simulink model "HVDC_MMC1_EMT"  (R2023b)
settings: Solver=ode23tb  StartTime=0.0  StopTime=10  MaxStep=Ts  RelTol=1e-3  EnableMultiTasking=on
PreLoadFcn:
  | HVDC_MMC_param
StartFcn:
  | tic
StopFcn:
  | toc
values from neighbouring files (symbols this model uses):
  acdcV = 1/(Vnom_dc/2*sqrt(3)/sqrt(2)/Vnom_sec)    [HVDC_MMC_param.m]
  C_PM = 1.758e-3    (= 0.001758)    [HVDC_MMC_param.m]
  Carm = 1.0*C_pm/n    (= 0.0002096)    [B2B_HVDC_MMC_Calc.m]    (also in HVDC_MMC_param.m = 4.88333333333e-05)
  DC_cable_C_shunt = 0.1e-6    (= 1e-07)    [HVDC_MMC_param.m]
  DC_cable_R_shunt = 1000    [HVDC_MMC_param.m]
  DCM = 1    [HVDC_MMC_param.m]
  Fn_filter = 1000    [B2B_HVDC_MMC_Calc.m]    (also in HVDC_MMC_param.m)
  Fnom = 50    [HVDC_MMC_param.m]
  HRM = 2    [HVDC_MMC_param.m]
  HrmOrd = N    (= 2)    [B2B_HVDC_MMC_Calc.m]    (also in HVDC_MMC_param.m)
  Ib_ac = (2/3)*Pnom/Vb_ac    [HVDC_MMC_param.m]
  Ib_dc = Pnom/Vb_dc    (= 1501.5015015)    [HVDC_MMC_param.m]
  Ki_CCSC = 50    [HVDC_MMC_param.m]
  Ki_Ireg = 6    [HVDC_MMC_param.m]
  Ki_Preg = 1.0    (= 1)    [HVDC_MMC_param.m]
  Ki_Qreg = 1.0    (= 1)    [HVDC_MMC_param.m]
  Ki_VDCreg = 100    [HVDC_MMC_param.m]
  Kp_CCSC = 0.8    [HVDC_MMC_param.m]
  Kp_Ireg = 0.6    [HVDC_MMC_param.m]
  Kp_Preg = 0.5/3    (= 0.166666666667)    [HVDC_MMC_param.m]
  Kp_Qreg = 0.5/3    (= 0.166666666667)    [HVDC_MMC_param.m]
  Kp_VDCreg = 4    [HVDC_MMC_param.m]
  L_cable = 15e-3    (= 0.015)    [HVDC_MMC_param.m]
  Larm = Larm_pu*(Zb_ac/w)    [HVDC_MMC_param.m]
  Lff = Larm_pu/2+Lxfo    (= 0.195)    [HVDC_MMC_param.m]
  Limits_Ireg = [ 2.0  -2.0]    [HVDC_MMC_param.m]
  Limits_Preg = [ 1.2, 0.8 ]    [HVDC_MMC_param.m]
  Limits_Qreg = [ 0.25, -0.25 ]    [HVDC_MMC_param.m]
  Limits_VDCreg = [ 2.0  -2.0]    [HVDC_MMC_param.m]
  Lxfo = 0.12    [HVDC_MMC_param.m]
  Pac = 0.9    [HVDC_MMC_param.m]
  Pnom = 1000e6    (= 1000000000)    [HVDC_MMC_param.m]
  Qac = 0.2    [HVDC_MMC_param.m]
  QCM = 0    [HVDC_MMC_param.m]
  R_cable = 0.5    [HVDC_MMC_param.m]
  Rarm = Rarm_pu*Zb_ac    [HVDC_MMC_param.m]
  Rff = Rarm_pu/2+Rxfo    (= 0.00375)    [HVDC_MMC_param.m]
  Rxfo = 0.003    [HVDC_MMC_param.m]
  Slope_Pref = 0.5    [HVDC_MMC_param.m]
  Slope_Qref = 0.5    [HVDC_MMC_param.m]
  Slope_Vdc_ref = Vnom_dc/5    (= 133200)    [HVDC_MMC_param.m]
  Tbrk1_On = 0.1    [HVDC_MMC_param.m]
  Tbrk2_On = 1.0    (= 1)    [HVDC_MMC_param.m]
  Tdeblock = 1.5    [HVDC_MMC_param.m]
  Tfault = 9999    [HVDC_MMC_param.m]
  Ton_Converter2 = 3    [HVDC_MMC_param.m]
  Ton_PQreg = 2    [HVDC_MMC_param.m]
  Ton_VDCreg = 1.5    [HVDC_MMC_param.m]
  Ts = Ts_Power    (= 5e-05)    [B2B_HVDC_MMC_Calc.m]    (also in HVDC_MMC_param.m)
  Ts_Control = Ts_Power    (= 5e-05)    [B2B_HVDC_MMC_Calc.m]    (also in HVDC_MMC_param.m)
  Ts_DQN = MultTs*Ts_Power    (= 5e-05)    [B2B_HVDC_MMC_Calc.m]    (also in HVDC_MMC_param.m)
  Ts_EMT = Ts    (= 5e-05)    [HVDC_MMC_param.m]
  Ts_Power = 1*50e-6    (= 5e-05)    [B2B_HVDC_MMC_Calc.m]    (also in HVDC_MMC_param.m)
  Vb_ac = sqrt(2/3)*Vnom_sec    [HVDC_MMC_param.m]
  Vb_dc = Vnom_dc    (= 666000)    [HVDC_MMC_param.m]
  Vc0_PM = 0    [HVDC_MMC_param.m]
  Vnom_dc = 2*Vnom_sec    (= 666000)    [HVDC_MMC_param.m]
  Vnom_prim = 333e3    (= 333000)    [HVDC_MMC_param.m]
  Vnom_sec = 333e3    (= 333000)    [HVDC_MMC_param.m]
  w = 2*pi*f    (= 314.159265359)    [B2B_HVDC_MMC_Calc.m]    (also in HVDC_MMC_param.m)
  Ws = 2*pi*Fnom    (= 314.159265359)    [HVDC_MMC_param.m]
  Zb_ac = Vb_ac/Ib_ac    [HVDC_MMC_param.m]
  Zeta_filter = 1    [B2B_HVDC_MMC_Calc.m]    (also in HVDC_MMC_param.m)
undefined symbols (not defined in the file or in its folder): DCss, DiscIntNeverNeededParam, gcbh, MT, sps_rtmsupport
libraries: DQN_Lib x37, simulink x35, spsCurrentMeasurementLib x24, powerlib_extras x21, slpidlib x14, spsSecondOrderFilterLib x14, spsVoltageMeasurementLib x10, spsSeriesRLCBranchLib x10, spsControlledVoltageSourceLib x9, spsHalfBridgeMMCmodel x7, spsGroundLib x4, spsParallelRLCBranchLib x4
(part 3 of 9)

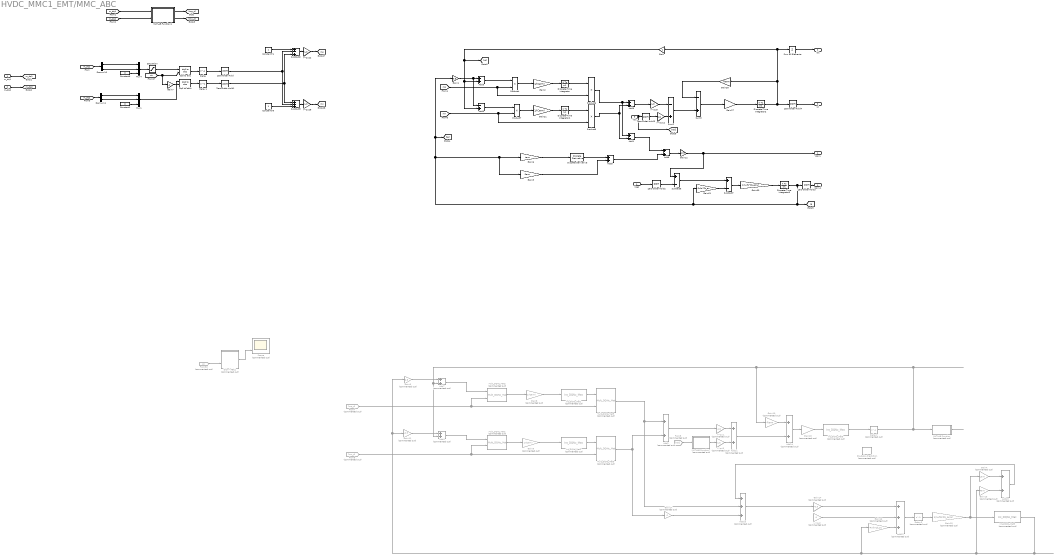
== system HVDC_MMC1_EMT/MMC_ABC ==
  m_dq1 : Inport
  m_dq2 : Inport  Port=2
  Vdc : Inport  Port=3
  Vsec : Inport  Port=4
  Add1 : Sum  Inputs=+-
  Add10 : Sum  Commented=on  Inputs=+++
  Add{2,4,7,11,13..14} (6 alike) : Sum  Commented=on
  Add12 : Sum  Commented=on  Inputs=+++
  Add{3,5,8..9} (4 alike) : Sum
  Add6 : Sum  Inputs=-+
  Constant1 : Constant  Value=0
  Constant6 : Constant  Value=0
  Constant74 : Constant
  Constant75 : Constant
  DQn->ABC1 : MATLAB Function  Commented=on  TreatAsAtomicUnit=on  SystemSampleTime=Ts  mask{N=HrmOrd}
      mask prompts: N "Harmonic order:"
  Delay : Delay  DelayLength=1
  Delay1 : Delay  DelayLength=1
  Delay2 : Delay  Commented=on  DelayLength=1  SampleTime=Ts
  Delay3 : Delay  Commented=on  DelayLength=1  SampleTime=Ts
  Demux10 : Demux  Outputs=2
  Demux11 : Demux  Outputs=2
  Discrete Derivative : simulink/Discrete/Discrete Derivative  gainval=1.0  ICPrevScaledInput=0.0  OutMin=[]  OutMax=[]  OutDataType=fixdt(1, 16)  OutScaling=2^-10  DoSatur=off
  Discrete-Time Integrator{,1..3} (4 alike) : DiscreteIntegrator  SampleTime=Ts_EMT  ICPrevOutput=DiscIntNeverNeededParam  ICPrevScaledInput=DiscIntNeverNeededParam
  From30 : From  Commented=on  GotoTag=wt  TagVisibility=global
  From5 : From  Commented=on  GotoTag=Vdc
  From7 : From  Commented=on  GotoTag=mp_c
  From8 : From  Commented=on  GotoTag=mn_c
  Gain : Gain
  Gain1 : Gain  Gain=0.5
  Gain10 : Gain  Commented=on  Gain=-Rarm
  Gain11 : Gain  Commented=on  Gain=-0.5
  Gain12 : Gain  Gain=-0.5
  Gain13 : Gain  Commented=on  Gain=Rarm
  Gain14 : Gain  Commented=on  Gain=-0.5
  Gain15 : Gain  Commented=on  Gain=1/(Lxfo*Zb_ac/w)
  Gain16 : Gain  Commented=on  Gain=-Rxfo*Zb_ac
  Gain17 : Gain  Commented=on  Gain=-1
  Gain18 : Gain  Commented=on  Gain=1/(Larm)
  Gain2 : Gain  Gain=1/(Carm)
  Gain21 : Gain  Gain=1/(Carm)
  Gain27 : Gain  Gain=1/(Larm)
  Gain28 : Gain  Gain=Rarm
  Gain3 : Gain  Gain=Rarm
  Gain4 : Gain  Commented=on  Gain=Larm
  Gain5 : Gain  Commented=on  Gain=0.5
  Gain6 : Gain  Gain=Larm
  Gain60 : Gain  Gain=1/(Lxfo*Zb_ac/w)
  Gain61 : Gain  Gain=Rxfo*Zb_ac
  Gain7 : Gain  Gain=-2
  Gain8 : Gain  Commented=on  Gain=1/(Carm)
  Gain9 : Gain  Commented=on  Gain=1/(Carm)
  I->pu1 : Gain  Commented=on  Gain=-1/2  SaturateOnIntegerOverflow=on  OutDataTypeStr=Inherit: Same as input  ParamDataTypeStr=Inherit: Same as input
  I->pu{5,12,22,28} (4 alike) : Gain  Gain=1/2  SaturateOnIntegerOverflow=on  OutDataTypeStr=Inherit: Same as input  ParamDataTypeStr=Inherit: Same as input
  I->pu2 : Gain  Commented=on  Gain=-1  SaturateOnIntegerOverflow=on  OutDataTypeStr=Inherit: Same as input  ParamDataTypeStr=Inherit: Same as input
  I->pu3 : Gain  Commented=on  Gain=1/2  SaturateOnIntegerOverflow=on  OutDataTypeStr=Inherit: Same as input  ParamDataTypeStr=Inherit: Same as input
  Int_DQNc_Mat{1..3,5} (4 alike) : DQN_Lib/Int_DQNc_Mat  Commented=on  N=HrmOrd  dt=Ts  w=Ws  InitInt=0*[0.8; 0.6; -0.33]  swFeed=off  R=1  iL=1
  MATLAB Function : MATLAB Function  Commented=on  TreatAsAtomicUnit=on
  MATLAB Function1 : MATLAB Function  TreatAsAtomicUnit=on  mask{N=HrmOrd}
      mask prompts: N "Harmonic order:"
  MATLAB Function2 : MATLAB Function  Commented=on  TreatAsAtomicUnit=on  mask{N=HrmOrd}
      mask prompts: N "Harmonic order:"
  Mult_DQNc_Mat{1..3,5} (4 alike) : DQN_Lib/Mult_DQNc_Mat  Commented=on  N=HrmOrd  HrmDbl=off
  Mux1 : Mux  Inputs=3
  Mux4 : Mux  Inputs=3
  Product{4,6..8} (4 alike) : Product
  SS_DelayPrediction : DQN_Lib/SS_DelayPrediction  Commented=on  N=HrmOrd  Ts=Ts  x0=zeros(3,1)
  Saturation : Saturate  UpperLimit=Limits_Ireg(1)  LowerLimit=Limits_Ireg(2)
  Scope : Scope  Commented=on  NumInputPorts=2
  Subtract2 : Sum  Inputs=+-+
  Subtract5 : Sum  Inputs=+++
  Subtract6 : Sum  Inputs=+-
  Subtract7 : Sum  Inputs=+-
  Sum of Elements : Sum  Inputs=+
  Sum2 : Sum  Inputs=-+  InputSameDT=on  SaturateOnIntegerOverflow=on  OutDataTypeStr=Inherit: Same as first input
  Sum3 : Sum  Inputs=-+  InputSameDT=on  SaturateOnIntegerOverflow=on  OutDataTypeStr=Inherit: Same as first input
  Zero-Order Hold{,1..3} (4 alike) : ZeroOrderHold  SampleTime=Ts_EMT
  Zero-Order Hold4 : ZeroOrderHold  SampleTime=Ts
  Zero-Order Hold5 : ZeroOrderHold  SampleTime=Ts
  dq0 to abc : spsdq0toabcLib/dq0 to abc  Alignment=90 degrees behind phase A axis
  dq0 to abc1 : spsdq0toabcLib/dq0 to abc  Alignment=90 degrees behind phase A axis
  Vconv : Outport
  Idc : Outport  Port=2
  Id : Outport  Port=3
  Iconv1 : Outport  Port=4  VectorParamsAs1DForOutWhenUnconnected=off
  tag scope: Ig=global, m_dq1=global, m_dq2=global, mn=global, mp=global
  wires:
  Gain21/1 -> Discrete-Time Integrator1/1  "dVn_M"
  Add6/1 -> Product7/1
  Discrete-Time Integrator2/1 -> Zero-Order Hold4/1, Gain/1, Sum of Elements/1, Gain28/1  "dVp_M"
  Gain1/1 -> Add6/1, Add3/1
  Sum2/1 -> Sum3/2
  Add1/1 -> Add8/1
  Add3/1 -> Product4/1  "prod"
  Gain3/1 -> Add5/2  "dVp_M"
  Discrete-Time Integrator1/1 -> Product8/1  "Vn_M"
  Gain6/1 -> Discrete Derivative/1  "dVp_M"
  Discrete Derivative/1 -> Add5/1
  Gain28/1 -> Sum3/1
  Product8/1 -> Add9/2, Add1/2
  Add9/1 -> I->pu5/1  "dVp_M"
  Product7/1 -> Gain21/1
  Discrete-Time Integrator/1 -> Product6/1  "Vp_M"
  Add8/1 -> Gain12/1
  Gain2/1 -> Discrete-Time Integrator/1  "dVp_M"
  I->pu12/1 -> Sum2/2
  I->pu5/1 -> Sum2/1
  Sum3/1 -> Gain27/1
  Vdc/1 -> [Vdc], Zero-Order Hold3/1
  Gain12/1 -> Vconv/1, Subtract6/1  "prod"
  Add5/1 -> Add8/2
  Sum of Elements/1 -> Idc/1
  m_dq1/1 -> [m_dq1]
  m_dq2/1 -> [m_dq2]
  Gain/1 -> [Id], Add6/2, Add3/2
  Gain27/1 -> Discrete-Time Integrator2/1
  Subtract7/1 -> Gain60/1
  Vsec/1 -> Zero-Order Hold2/1
  Gain61/1 -> Subtract7/2
  Subtract6/1 -> Subtract7/1
  Gain60/1 -> Discrete-Time Integrator3/1
  Discrete-Time Integrator3/1 -> Zero-Order Hold5/1, [Ig], Gain1/1, Gain3/1, Gain6/1, Gain61/1, [Ig]  "Igd"
  I->pu22/1 -> [mp]
  Constant75/1 -> Subtract5/3
  Subtract2/1 -> I->pu22/1
  Constant74/1 -> Subtract2/1
  Delay1/1 -> Zero-Order Hold1/1
  [m_dq2] -> Demux11/1
  [m_dq1] -> Demux10/1
  Demux10/2 -> Mux4/2
  Gain7/1 -> dq0 to abc1/2
  I->pu28/1 -> [mn]
  Demux10/1 -> Mux4/1
  Mux1/1 -> dq0 to abc1/1
  Constant6/1 -> Mux4/3
  Mux4/1 -> Saturation/1
  Delay/1 -> Zero-Order Hold/1
  Demux11/2 -> Mux1/2
  Subtract5/1 -> I->pu28/1
  dq0 to abc1/1 -> Delay1/1
  dq0 to abc/1 -> Delay/1
  [wt] -> Gain7/1, dq0 to abc/2
  Saturation/1 -> dq0 to abc/1
  Demux11/1 -> Mux1/1
  Constant1/1 -> Mux1/3
  [mp] -> Product6/2, Product4/2
  [mn] -> Product8/2, Product7/2
  Zero-Order Hold/1 -> Subtract5/2, Subtract2/2
  Zero-Order Hold1/1 -> Subtract5/1, Subtract2/3
  Zero-Order Hold2/1 -> Subtract6/2
  Zero-Order Hold3/1 -> I->pu12/1
  Zero-Order Hold4/1 -> Id/1
  Zero-Order Hold5/1 -> Iconv1/1
  Product6/1 -> Add1/1, Add9/1  "Iabc_B22 (A)"
  Product4/1 -> Gain2/1
  Gain14/1 -> Add12/1
  Gain17/1 -> Add10/3
  Add13/1 -> Add10/1
  Mult_DQNc_Mat5/1 -> Add2/1, Add10/2
  Add11/1 -> Add14/2
  Mult_DQNc_Mat2/1 -> Gain8/1
  Gain4/1 -> Add13/1  "dVp_M"
  Gain9/1 -> Int_DQNc_Mat2/1
  I->pu2/1 -> Add12/2
  [m_dq1] -> MATLAB Function1/1(m1_dq)
  From8/1 -> Mult_DQNc_Mat3/2, Mult_DQNc_Mat1/2
  ? -> I->pu2/1
  Gain16/1 -> Add12/3
  I->pu1/1 -> Add11/1
  Add10/1 -> Gain14/1
  Mult_DQNc_Mat1/1 -> Gain9/1
  MATLAB Function/1(y) -> ?
  Mult_DQNc_Mat3/1 -> Gain17/1, Add2/2
  Gain10/1 -> Add14/1
  Gain18/1 -> Int_DQNc_Mat3/1
  Gain15/1 -> Int_DQNc_Mat5/1, Gain4/1
  Add7/1 -> Mult_DQNc_Mat2/1
  Add14/1 -> Gain18/1
  MATLAB Function2/1(Vdc_c) -> I->pu3/1
  Delay3/1 -> Gain15/1
  Int_DQNc_Mat3/1 -> Delay2/1  "dw"
  Gain8/1 -> Int_DQNc_Mat1/1
  Add2/1 -> I->pu1/1
  Int_DQNc_Mat5/1 -> Gain5/1, Gain11/1, Gain16/1, Gain13/1
  Add12/1 -> Delay3/1
  From7/1 -> Mult_DQNc_Mat5/2, Mult_DQNc_Mat2/2
  Int_DQNc_Mat1/1 -> Mult_DQNc_Mat5/1
  Gain11/1 -> Add4/1
  MATLAB Function1/1(mp_c) -> [mp_c]
  Gain13/1 -> Add13/2
  Gain5/1 -> Add7/1
  I->pu3/1 -> Add11/2
  MATLAB Function1/2(mn_c) -> [mn_c]
  [m_dq2] -> MATLAB Function1/2(m2_dq)
  Add4/1 -> Mult_DQNc_Mat1/1
  Int_DQNc_Mat2/1 -> Mult_DQNc_Mat3/1
  From5/1 -> MATLAB Function2/1(Vdc)
  Delay2/1 -> MATLAB Function/1(u), Add4/2, Add7/2, Gain10/1
  From30/1 -> DQn->ABC1/2(tho)
  DQn->ABC1/1(Xabc) -> Scope/2

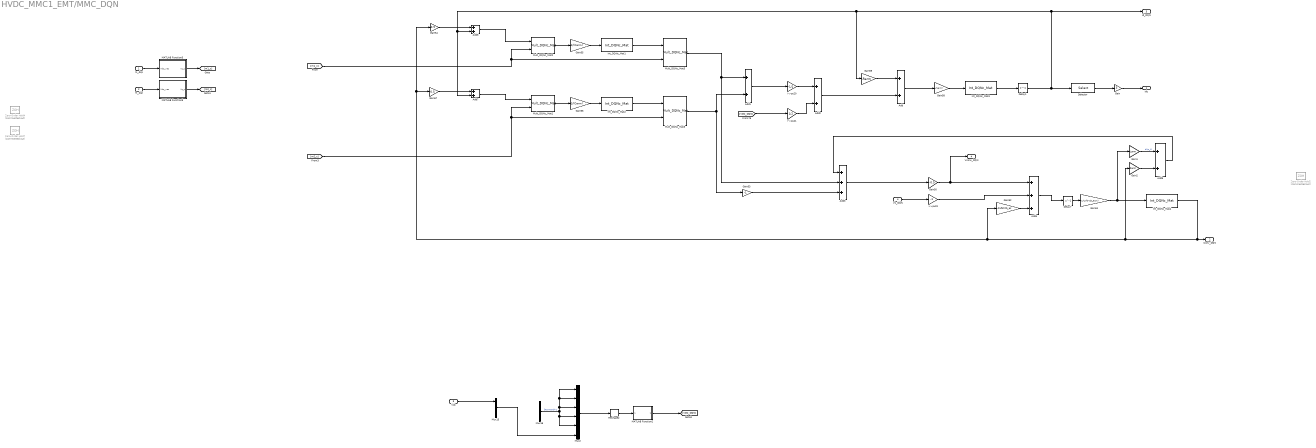
== system HVDC_MMC1_EMT/MMC_DQN ==
  m_dq1 : Inport
  m_dq2 : Inport  Port=2
  Vdc : Inport  Port=3
  Vs_DQN : Inport  Port=4
  Add{,1..2,5..7} (6 alike) : Sum
  Add3 : Sum  Inputs=+++
  Add4 : Sum  Inputs=+++
  Delay1 : Delay  DelayLength=1  SampleTime=TimeStep
  Delay7 : Delay  DelayLength=1  SampleTime=TimeStep
  Gain : Gain  Gain=3
  Gain1 : Gain  Gain=Larm
  Gain2 : Gain  Gain=Rarm
  Gain50 : Gain  Gain=-0.5
  Gain51 : Gain  Gain=1/(Lxfo*Zb_ac/w)
  Gain52 : Gain  Gain=-Rxfo*Zb_ac
  Gain53 : Gain  Gain=-1
  Gain54 : Gain  Gain=0.5
  Gain55 : Gain  Gain=1/(Carm)
  Gain56 : Gain  Gain=1/(Carm)
  Gain57 : Gain  Gain=-0.5
  Gain58 : Gain  Gain=1/(Larm)
  Gain59 : Gain  Gain=-Rarm
  I->pu20 : Gain  Gain=-1/2  SaturateOnIntegerOverflow=on  OutDataTypeStr=Inherit: Same as input  ParamDataTypeStr=Inherit: Same as input
  I->pu21 : Gain  Gain=1/2  SaturateOnIntegerOverflow=on  OutDataTypeStr=Inherit: Same as input  ParamDataTypeStr=Inherit: Same as input
  I->pu23 : Gain  Gain=-1  SaturateOnIntegerOverflow=on  OutDataTypeStr=Inherit: Same as input  ParamDataTypeStr=Inherit: Same as input
  Int_DQNc_Mat{1..4} (4 alike) : DQN_Lib/Int_DQNc_Mat  N=HrmOrd  dt=TimeStep  w=AngFreq  InitInt=0*[0.8; 0.6; -0.33]  swFeed=off  R=1  iL=1
  MATLAB Function2 : MATLAB Function  TreatAsAtomicUnit=on
  MATLAB Function3 : MATLAB Function  TreatAsAtomicUnit=on  mask{N=HrmOrd}
      mask prompts: N "Harmonic order:"
  MATLAB Function5 : MATLAB Function  TreatAsAtomicUnit=on  mask{N=HrmOrd}
      mask prompts: N "Harmonic order:"
  Mult_DQNc_Mat{1..3,5} (4 alike) : DQN_Lib/Mult_DQNc_Mat  N=HrmOrd  HrmDbl=off
  Mux15 : Mux  Inputs=HrmOrd+1
  Mux16 : Mux  Inputs=HrmOrd+1
  Mux2 : Mux  Inputs=[HrmOrd+1, HrmOrd+1, HrmOrd+1, HrmOrd+1, HrmOrd+1, HrmOrd+1]
  Reshape2 : Reshape  OutputDimensionality=Customize  OutputDimensions=[HRM+1,6]
  Selector : Selector  InputPortWidth=6*(HRM+1)  IndexOptions=Index vector (dialog)  Indices=5*(HRM+1)+1  OutputSizes=1
  Zero-Order Hold2 : ZeroOrderHold  Commented=on  SampleTime=Ts_DQN
  Zero-Order Hold4 : ZeroOrderHold  Commented=on  SampleTime=TimeStep
  Zero-Order Hold7 : ZeroOrderHold  Commented=on  SampleTime=TimeStep
  Idc : Outport
  Iconv_DQN : Outport  Port=2  VectorParamsAs1DForOutWhenUnconnected=off
  Id_DQN : Outport  Port=3
  Vconv_DQN : Outport  Port=4  VectorParamsAs1DForOutWhenUnconnected=off
  wires:
  Add/1 -> Gain58/1
  Gain58/1 -> Int_DQNc_Mat3/1
  Mux15/1 -> Mux2/6
  [VDC_DQN] -> I->pu21/1
  Gain57/1 -> Add7/1
  Mult_DQNc_Mat1/1 -> Gain56/1
  Gain54/1 -> Add6/1
  Mux16/1 -> Mux2/3, Mux2/2, Mux2/1, Mux2/4, Mux2/5  "[HarmOrd+1"
  I->pu20/1 -> Add2/1
  Gain59/1 -> Add/1
  Gain/1 -> Idc/1
  Selector/1 -> Gain/1
  Mult_DQNc_Mat2/1 -> Gain55/1
  Gain52/1 -> Add4/3
  Gain50/1 -> Add4/1, Vconv_DQN/1
  Gain1/1 -> Add5/1  "dVp_M"
  Gain2/1 -> Add5/2
  Add5/1 -> Add3/1
  Gain51/1 -> Int_DQNc_Mat4/1, Gain1/1
  Add4/1 -> Delay7/1
  Delay7/1 -> Gain51/1
  Gain55/1 -> Int_DQNc_Mat1/1
  Gain56/1 -> Int_DQNc_Mat2/1
  I->pu23/1 -> Add4/2
  I->pu21/1 -> Add2/2
  Add1/1 -> I->pu20/1
  Vdc/1 -> Mux15/1
  Add2/1 -> Add/2
  Gain53/1 -> Add3/3
  Add3/1 -> Gain50/1
  [m1_c] -> Mult_DQNc_Mat5/2, Mult_DQNc_Mat2/2
  [m2_c] -> Mult_DQNc_Mat3/2, Mult_DQNc_Mat1/2
  Int_DQNc_Mat3/1 -> Delay1/1
  Int_DQNc_Mat1/1 -> Mult_DQNc_Mat5/1
  Int_DQNc_Mat2/1 -> Mult_DQNc_Mat3/1
  Add6/1 -> Mult_DQNc_Mat2/1
  Add7/1 -> Mult_DQNc_Mat1/1
  Mult_DQNc_Mat3/1 -> Gain53/1, Add1/2
  Mult_DQNc_Mat5/1 -> Add3/2, Add1/1
  Int_DQNc_Mat4/1 -> Gain54/1, Gain57/1, Gain52/1, Gain2/1, Iconv_DQN/1
  Vs_DQN/1 -> I->pu23/1
  Delay1/1 -> Selector/1, Add7/2, Add6/2, Gain59/1, Id_DQN/1
  Reshape2/1 -> MATLAB Function2/1(X_DQN)
  Mux2/1 -> Reshape2/1
  MATLAB Function2/1(Ydcpnz_c) -> [VDC_DQN]
  MATLAB Function3/1(Vs_c) -> [m1_c]
  MATLAB Function5/1(Vs_c) -> [m2_c]
  m_dq2/1 -> MATLAB Function5/1(Vdq_vec)
  m_dq1/1 -> MATLAB Function3/1(Vdq_vec)

== system HVDC_MMC1_EMT/MMC_DQN1 ==
  m_dq1 : Inport
  m_dq2 : Inport  Port=2
  Vdc : Inport  Port=3
  Vs_DQN : Inport  Port=4
  Add10 : Sum  Inputs=+++
  Add{6..9,11,13} (6 alike) : Sum
  Add12 : Sum  Inputs=+++
  Delay : Delay  DelayLength=1  SampleTime=Ts
  Delay2 : Delay  DelayLength=1  SampleTime=TimeStep
  Gain10 : Gain  Gain=-Rarm
  Gain12 : Gain  Gain=Larm
  Gain13 : Gain  Gain=Rarm
  Gain14 : Gain  Gain=-0.5
  Gain15 : Gain  Gain=1/(Lxfo*Zb_ac/w)
  Gain16 : Gain  Gain=-Rxfo*Zb_ac
  Gain17 : Gain  Gain=-1
  Gain3 : Gain  Gain=0.5
  Gain6 : Gain  Gain=1/(Carm)
  Gain7 : Gain  Gain=1/(Carm)
  Gain8 : Gain  Gain=-0.5
  Gain9 : Gain  Gain=1/(Larm)
  I->pu1 : Gain  Gain=-1/2  SaturateOnIntegerOverflow=on  OutDataTypeStr=Inherit: Same as input  ParamDataTypeStr=Inherit: Same as input
  I->pu3 : Gain  Gain=1/2  SaturateOnIntegerOverflow=on  OutDataTypeStr=Inherit: Same as input  ParamDataTypeStr=Inherit: Same as input
  I->pu5 : Gain  Gain=-1  SaturateOnIntegerOverflow=on  OutDataTypeStr=Inherit: Same as input  ParamDataTypeStr=Inherit: Same as input
  Int_DQNc_Mat{1..4} (4 alike) : DQN_Lib/Int_DQNc_Mat  N=HrmOrd  dt=TimeStep  w=AngFreq  InitInt=0*[0.8; 0.6; -0.33]  swFeed=off  R=1  iL=1
  MATLAB Function : MATLAB Function  TreatAsAtomicUnit=on
  MATLAB Function1 : MATLAB Function  TreatAsAtomicUnit=on  mask{N=HrmOrd}
      mask prompts: N "Harmonic order:"
  MATLAB Function4 : MATLAB Function  TreatAsAtomicUnit=on  mask{N=HrmOrd}
      mask prompts: N "Harmonic order:"
  Mult_DQNc_Mat{1..3,5} (4 alike) : DQN_Lib/Mult_DQNc_Mat  N=HrmOrd  HrmDbl=off
  SS_DelayPrediction : DQN_Lib/SS_DelayPrediction  Commented=on  N=HrmOrd  Ts=Ts  x0=zeros(3,1)
  Zero-Order Hold4 : ZeroOrderHold  Commented=on  SampleTime=TimeStep
  Zero-Order Hold7 : ZeroOrderHold  Commented=on  SampleTime=TimeStep
  Idc : Outport
  Iconv_DQN : Outport  Port=2  VectorParamsAs1DForOutWhenUnconnected=off
  Id_DQN : Outport  Port=3
  wires:
  Vdc/1 -> MATLAB Function4/1(Vdc)
  m_dq2/1 -> MATLAB Function1/2(m2_dq)
  MATLAB Function1/1(mp_c) -> [mp_c]
  MATLAB Function1/2(mn_c) -> [mn_c]
  [mn_c] -> Mult_DQNc_Mat3/2, Mult_DQNc_Mat1/2
  Mult_DQNc_Mat2/1 -> Gain6/1
  Gain3/1 -> Add7/1
  Int_DQNc_Mat4/1 -> Iconv_DQN/1, Gain3/1, Gain8/1, Gain16/1, Gain13/1
  Mult_DQNc_Mat1/1 -> Gain7/1
  Int_DQNc_Mat1/1 -> Mult_DQNc_Mat5/1
  Add8/1 -> Mult_DQNc_Mat1/1
  Int_DQNc_Mat2/1 -> Mult_DQNc_Mat3/1
  [mp_c] -> Mult_DQNc_Mat5/2, Mult_DQNc_Mat2/2
  Gain6/1 -> Int_DQNc_Mat1/1
  Add7/1 -> Mult_DQNc_Mat2/1
  Gain8/1 -> Add8/1
  Gain7/1 -> Int_DQNc_Mat2/1
  I->pu3/1 -> Add11/2
  I->pu1/1 -> Add11/1
  MATLAB Function4/1(Vdc_c) -> I->pu3/1
  Add6/1 -> I->pu1/1
  Gain10/1 -> Add9/1
  Gain9/1 -> Int_DQNc_Mat3/1
  Add9/1 -> Gain9/1
  Add11/1 -> Add9/2
  m_dq1/1 -> MATLAB Function1/1(m1_dq)
  Int_DQNc_Mat3/1 -> Delay/1  "dw"
  Delay/1 -> MATLAB Function/1(u), Add8/2, Add7/2, Gain10/1, Id_DQN/1
  Gain12/1 -> Add13/1  "dVp_M"
  Mult_DQNc_Mat3/1 -> Gain17/1, Add6/2
  I->pu5/1 -> Add12/2
  Add13/1 -> Add10/1
  Add10/1 -> Gain14/1
  Mult_DQNc_Mat5/1 -> Add6/1, Add10/2
  Add12/1 -> Delay2/1
  Vs_DQN/1 -> I->pu5/1
  Gain16/1 -> Add12/3
  Delay2/1 -> Gain15/1
  Gain13/1 -> Add13/2
  Gain15/1 -> Int_DQNc_Mat4/1, Gain12/1
  Gain14/1 -> Add12/1
  Gain17/1 -> Add10/3
  MATLAB Function/1(y) -> Idc/1

== system HVDC_MMC1_EMT/Sequencer ==
  note: Open breaker 1 when a fault occur
  note: Block the converter when a fault occur
  note: Block the converter when a fault occur
  note: STEP 6: Reactive power regulator setpoint
  note: STEP 4: Enable PQ regulators and converter 2
  note: STEP 5: Active power regulator setpoint
  note: STEP 3 : Voltage regulator setpoint
  note: STEP 2 : Deblocking converter 1
  note: STEP 1 : Energization
  note: EXTRA STEP: Program a fault
  note: STEP 5: Active power regulator setpoint
  note: PSCC
  BL1 : Step  Time=Tbrk1_On  SampleTime=Ts_Power
  BL10 : Step  Time=Tfault+Ts_Power  SampleTime=Ts_Power
  BL11 : Step  Time=Tfault  SampleTime=Ts_Power
  BL2 : Step  Time=Tbrk2_On  SampleTime=Ts_Power
  BL3 : Step  Time=Ton_Converter2  SampleTime=Ts_Power
  BL4 : Step  Time=Ton_VDCreg  SampleTime=Ts
  BL5 : Step  Time=Tdeblock  Before=1  After=0  SampleTime=Ts_Power
  BL6 : Step  Time=Ton_PQreg  SampleTime=Ts
  BL7 : Step  Time=3  SampleTime=Ts_Power
  BL8 : Step  Time=Tfault + 1.95*(1/Fnom)  Before=1  After=0  SampleTime=Ts_Power
  BL9 : Step  Time=Tfault + 2*(1/Fnom)  Before=1  After=0  SampleTime=Ts_Power
  Logical Operator : Logic  AllPortsSameDT=off  OutDataTypeStr=boolean
  Logical Operator1 : Logic  Operator=OR  AllPortsSameDT=off  OutDataTypeStr=float('double')
  Logical Operator2 : Logic  AllPortsSameDT=off  OutDataTypeStr=boolean
  Pref : simulink/Sources/Ramp  slope=Slope_Pref*sign(Pac)  start=Tramping_Pref  InitialOutput=0
  Pref1 : simulink/Sources/Ramp  slope=1  start=0.5  InitialOutput=0
  Product : Product
  Product1 : Product  Inputs=3
  Qref : simulink/Sources/Ramp  slope=Slope_Qref*sign(Qac)  start=Tramping_Qref  InitialOutput=0
  Rtot_pu2 : Gain  Gain=1/Vnom_dc  SaturateOnIntegerOverflow=on  OutDataTypeStr=Inherit: Same as input  ParamDataTypeStr=Inherit: Same as input
  Saturation : Saturate  UpperLimit=abs(Pac)  LowerLimit=-abs(Pac)
  Saturation1 : Saturate  UpperLimit=abs(Qac)  LowerLimit=-abs(Qac)
  Saturation2 : Saturate  UpperLimit=Vnom_dc  LowerLimit=eps
  Saturation3 : Saturate  UpperLimit=abs(Pac)  LowerLimit=-abs(Pac)
  Step : Step  Time=22  Before=1  After=1.05  SampleTime=0
  Step1 : Step  Time=3  Before=1  After=0.98  SampleTime=0
  Step2 : Step  Time=5  Before=1  After=1.02/0.98  SampleTime=0
  "Vdc_ref " : simulink/Sources/Ramp  slope=Slope_Vdc_ref  start=Tramping_Vdc_ref  InitialOutput=Vnom_sec*1.37
  tag scope: Blk=global, Brk1_On=global, Brk2_On=global, Converter2_On=global, Fault_On=global, PQreg_On=global, PSCC_On=global, Pac_ref=global, Qac_ref=global, VDCreg_On=global, Vdc_ref=global, Vdcx_ref=global
  wires:
  Pref/1 -> Saturation/1
  Qref/1 -> Saturation1/1
  Saturation/1 -> Product/1
  Saturation1/1 -> [Qac_ref]
  BL4/1 -> [VDCreg_On]
  BL6/1 -> [PQreg_On]
  "Vdc_ref "/1 -> Saturation2/1
  BL2/1 -> [Brk2_On]
  BL8/1 -> Logical Operator/2
  Logical Operator/1 -> [Brk1_On]
  BL1/1 -> Logical Operator/1
  BL9/1 -> Logical Operator2/2
  BL3/1 -> Logical Operator2/1
  Logical Operator2/1 -> [Converter2_On]
  Logical Operator1/1 -> [Blk]
  BL5/1 -> Logical Operator1/1
  BL10/1 -> Logical Operator1/2
  BL11/1 -> [Fault_On]
  Rtot_pu2/1 -> [Vdc_ref]
  Product/1 -> [Pac_ref]
  Step/1 -> Product/2
  Product1/1 -> [Vdcx_ref]
  Saturation3/1 -> Product1/1
  Step1/1 -> Product1/2
  Pref1/1 -> Saturation3/1
  Step2/1 -> Product1/3
  BL7/1 -> [PSCC_On]
  Saturation2/1 -> Rtot_pu2/1

== system HVDC_MMC1_EMT/Subsystem ==
  wt : Inport
  Vdc : Inport  Port=2
  Vsec : Inport  Port=3
  Idiff : Inport  Port=4
  Iconv : Inport  Port=5
  Gain9 : Gain  Gain=-2
  I->pu2 : Gain  Gain=1/Ib_ac  SaturateOnIntegerOverflow=on  OutDataTypeStr=Inherit: Same as input  ParamDataTypeStr=Inherit: Same as input
  I->pu4 : Gain  Gain=1/Ib_ac  SaturateOnIntegerOverflow=on  OutDataTypeStr=Inherit: Same as input  ParamDataTypeStr=Inherit: Same as input
  I->pu9 : Gain  Gain=1/Vb_ac  SaturateOnIntegerOverflow=on  OutDataTypeStr=Inherit: Same as input  ParamDataTypeStr=Inherit: Same as input
  Park Transform4 : eeTransforms/Park Transform  AxisAlignment=Q-axis  PowerInvariant=off
  Selector2 : Selector  InputPortWidth=3  IndexOptions=Index vector (dialog)  Indices=[1 2]  OutputSizes=1
  Selector4 : Selector  InputPortWidth=3  IndexOptions=Index vector (dialog)  Indices=[1 2]  OutputSizes=1
  Selector5 : Selector  InputPortWidth=3  IndexOptions=Index vector (dialog)  Indices=[1 2]  OutputSizes=1
  Subsystem1 : Subsystem  Commented=on
  Subsystem2 : Subsystem  mask{Ts=Ts, Fnom=Fnom, acdcV=acdcV, Fn_filter=Fn_filter, Zeta_filter=Zeta_filter, Kp_Preg=Kp_Preg, Ki_Preg=Ki_Preg, Limits_Preg_1=Limits_Preg(1), Limits_Preg_2=Limits_Preg(2), Kp_Qreg=Kp_Qreg, Ki_Qreg=Ki_Qreg, Limits_Qreg_1=Limits_Qreg(1), Limits_Qreg_2=Limits_Qreg(2), Kp_VDCreg=Kp_VDCreg, Ki_VDCreg=Ki_VDCreg, Limits_VDCreg_1=Limits_VDCreg(1), Limits_VDCreg_2=Limits_VDCreg(2), Kp_Ireg=Kp_Ireg, Ki_Ireg=Ki_Ireg, Limits_Ireg=Limits_Ireg, Rff=Rff, Lff=Lff, Kp_CCSC=Kp_CCSC, Ki_CCSC=Ki_CCSC}
      mask prompts: Ts "Sample time:"; Fnom "Fundamental frequency (Hz):"; Fn_filter "Natural frequency fn (Hz):"; Zeta_filter "Damping ratio Zeta"; Kp_Preg "Proportional (P):"; Ki_Preg "Integral (I):"; Limits_Preg_1 "Upper limit:"; Limits_Preg_2 "Lower limit:"; Kp_Qreg "Proportional (P):"; Ki_Qreg "Integral (I):"; Limits_Qreg_1 "Upper limit:"; Limits_Qreg_2 "Lower limit:"; Kp_VDCreg "Proportional (P):"; Ki_VDCreg "Integral (I):"; Limits_VDCreg_1 "Upper limit:"; Limits_VDCreg_2 "Lower limit:"; Kp_Ireg "Proportional (P):"; Ki_Ireg "Integral (I):"; Limits_Ireg "Output limits:"; Kp_CCSC "Proportional (P):"; Ki_CCSC "Integral (I):"
      mask DialogControl Container6 Prompt: General
      mask DialogControl Container14 Prompt: Filter
      mask DialogControl Container14_copy Prompt: Active power regulator
      mask DialogControl Container14_copy_copy Prompt: Reactive power regulator
      mask DialogControl Container14_copy_copy_copy Prompt: DC voltage regulator
      mask DialogControl Container14_copy_copy_copy_copy Prompt: Current regulator
      mask DialogControl Container14_copy_copy_copy_copy_copy Prompt: CCSC
  V->pu2 : Gain  Gain=1/Vb_ac  SaturateOnIntegerOverflow=on  OutDataTypeStr=Inherit: Same as input  ParamDataTypeStr=Inherit: Same as input
  abc to dq0 : spsabctodq0Lib/abc to dq0  Alignment=90 degrees behind phase A axis
  abc to dq1 : spsabctodq0Lib/abc to dq0  Alignment=90 degrees behind phase A axis
  "{m_dq1}" : Outport  VectorParamsAs1DForOutWhenUnconnected=off
  "{m_dq2}" : Outport  Port=2  VectorParamsAs1DForOutWhenUnconnected=off
  wires:
  Subsystem2/1(m_dq1) -> "{m_dq1}"/1
  Vsec/1 -> V->pu2/1
  abc to dq1/1 -> Selector5/1
  Vdc/1 -> I->pu9/1
  Iconv/1 -> I->pu2/1
  I->pu2/1 -> abc to dq1/1
  Park Transform4/1 -> Selector2/1
  I->pu9/1 -> Subsystem2/1(Vdc)
  Gain9/1 -> Park Transform4/2
  wt/1 -> abc to dq0/2, abc to dq1/2, Gain9/1
  Subsystem2/2(m_dq2) -> "{m_dq2}"/1
  abc to dq0/1 -> Selector4/1
  Selector5/1 -> Subsystem2/3(Iconv_dq1)
  Selector4/1 -> Subsystem2/2(Vs_dq1)
  V->pu2/1 -> abc to dq0/1
  Idiff/1 -> I->pu4/1
  Selector2/1 -> Subsystem2/4(Id_dq2)
  I->pu4/1 -> Park Transform4/1
  [VDCreg_On] -> Subsystem2/6(VDCreg_On)
  [Vdc_ref] -> Subsystem2/7(Vdc_ref)
  [PSCC_On] -> Subsystem2/8(PQreg_On1)
  [PQreg_On] -> Subsystem2/5(PQreg_On)

== system HVDC_MMC1_EMT/Subsystem1 ==
  Constant16 : Constant  Value=DCM
  Constant2 : Constant  Value=DCM
  Controlled Voltage Source : spsControlledVoltageSourceLib/Controlled Voltage Source  Initialize=off  Source_Type=AC  Amplitude=0  Phase=0  Frequency=0  Measurements=None
  Controlled Voltage Source1 : spsControlledVoltageSourceLib/Controlled Voltage Source  Initialize=off  Source_Type=AC  Amplitude=0  Phase=0  Frequency=0  Measurements=None
  Current Measurement : spsCurrentMeasurementLib/Current Measurement  PhasorSimulation=off  OutputType=Complex  PSBequivalent=0
  Current Measurement1 : spsCurrentMeasurementLib/Current Measurement  PhasorSimulation=off  OutputType=Complex  PSBequivalent=0
  DC Voltage Regulator (VDCreg)1 : Subsystem
  Delay1 : Delay  DelayLength=1
  Gain2 : Gain
  Ground1 : spsGroundLib/Ground  LConnTagsString=a
  I->pu1 : Gain  Gain=Vnom_dc/2  SaturateOnIntegerOverflow=on  OutDataTypeStr=Inherit: Same as input  ParamDataTypeStr=Inherit: Same as input
  I->pu4 : Gain  Gain=1/Ib_dc  SaturateOnIntegerOverflow=on  OutDataTypeStr=Inherit: Same as input  ParamDataTypeStr=Inherit: Same as input
  I->pu9 : Gain  Gain=1/Vb_dc  SaturateOnIntegerOverflow=on  OutDataTypeStr=Inherit: Same as input  ParamDataTypeStr=Inherit: Same as input
  Multiply : Product
  PDC_ref1 : Step  Time=7  Before=0.8  After=0.75  SampleTime=0
  Switch1 : Switch  Criteria=u2 > Threshold  Threshold=0.5  OutDataTypeStr=double  SaturateOnIntegerOverflow=off  InputSameDT=off
  Switch3 : Switch  Criteria=u2 > Threshold  Threshold=0.5  OutDataTypeStr=double  SaturateOnIntegerOverflow=off  InputSameDT=off
  VDC_ref : Step  Time=13  Before=1  After=0.95  SampleTime=0
  Zcable1_3 : spsSeriesRLCBranchLib/Series RLC Branch  LConnTagsString=__new0  RConnTagsString=__new0  BranchType=RL  Resistance=R_cable/10  Inductance=L_cable/10  SetiL0=off  InitialCurrent=0  Capacitance=1e-6  Setx0=off  InitialVoltage=0  Measurements=None
  Zcable1_4 : spsSeriesRLCBranchLib/Series RLC Branch  LConnTagsString=__new0  RConnTagsString=__new0  BranchType=RL  Resistance=R_cable/10  Inductance=L_cable/10  SetiL0=off  InitialCurrent=0  Capacitance=1e-6  Setx0=off  InitialVoltage=0  Measurements=None
  REC2_plus : PMIOPort  Side=Left
  REC2_minus : PMIOPort  Port=2  Side=Left
  tag scope: Irec_minus=global, Irec_plus=global
  wires:
  PDC_ref1/1 -> Switch3/3
  Switch1/1 -> DC Voltage Regulator (VDCreg)1/2(Meas)
  Multiply/1 -> Switch1/3
  I->pu4/1 -> Multiply/2
  Switch3/1 -> DC Voltage Regulator (VDCreg)1/1(Ref)
  [Uctrl2] -> I->pu1/1
  I->pu9/1 -> Multiply/1, Switch1/1
  Gain2/1 -> [Uctrl2]
  [Idc1] -> I->pu4/1
  I->pu1/1 -> Controlled Voltage Source/1, Controlled Voltage Source1/1
  Constant16/1 -> Switch3/2
  VDC_ref/1 -> Switch3/1
  Constant2/1 -> Switch1/2
  Delay1/1 -> Gain2/1
  [Vdc2] -> I->pu9/1
  [Converter2_On] -> DC Voltage Regulator (VDCreg)1/3(On)
  DC Voltage Regulator (VDCreg)1/1(Id_ref) -> Delay1/1
  Current Measurement/1 -> [Irec_plus]
  Current Measurement1/1 -> [Irec_minus]
  connections:
  Controlled Voltage Source1/RConn1 -- Controlled Voltage Source/LConn1 -- Ground1/LConn1
  Controlled Voltage Source/RConn1 -- Zcable1_3/LConn1
  Controlled Voltage Source1/LConn1 -- Zcable1_4/LConn1
  Current Measurement/RConn1 -- Zcable1_3/RConn1
  Current Measurement/LConn1 -- REC2_plus/RConn1
  Zcable1_4/RConn1 -- Current Measurement1/RConn1
  Current Measurement1/LConn1 -- REC2_minus/RConn1

== system HVDC_MMC1_EMT/Subsystem2 ==
  Vsec : Inport
  Iconv : Inport  Port=2
  Vdc : Inport  Port=3
  wt : Inport  Port=4
  Idiff : Inport  Port=5
  Gain9 : Gain  Gain=-2
  I->pu2 : Gain  Gain=1/Ib_ac  SaturateOnIntegerOverflow=on  OutDataTypeStr=Inherit: Same as input  ParamDataTypeStr=Inherit: Same as input
  I->pu4 : Gain  Gain=1/Ib_ac  SaturateOnIntegerOverflow=on  OutDataTypeStr=Inherit: Same as input  ParamDataTypeStr=Inherit: Same as input
  I->pu9 : Gain  Gain=1/Vb_ac  SaturateOnIntegerOverflow=on  OutDataTypeStr=Inherit: Same as input  ParamDataTypeStr=Inherit: Same as input
  Park Transform4 : eeTransforms/Park Transform  AxisAlignment=Q-axis  PowerInvariant=off
  Selector2 : Selector  InputPortWidth=3  IndexOptions=Index vector (dialog)  Indices=[1 2]  OutputSizes=1
  Selector4 : Selector  InputPortWidth=3  IndexOptions=Index vector (dialog)  Indices=[1 2]  OutputSizes=1
  Selector5 : Selector  InputPortWidth=3  IndexOptions=Index vector (dialog)  Indices=[1 2]  OutputSizes=1
  Subsystem1 : Subsystem  mask{Ts=Ts, Fnom=Fnom, acdcV=acdcV, Fn_filter=Fn_filter, Zeta_filter=Zeta_filter, Kp_Preg=Kp_Preg, Ki_Preg=Ki_Preg, Limits_Preg_1=Limits_Preg(1), Limits_Preg_2=Limits_Preg(2), Kp_Qreg=Kp_Qreg, Ki_Qreg=Ki_Qreg, Limits_Qreg_1=Limits_Qreg(1), Limits_Qreg_2=Limits_Qreg(2), Kp_VDCreg=Kp_VDCreg, Ki_VDCreg=Ki_VDCreg, Limits_VDCreg_1=Limits_VDCreg(1), Limits_VDCreg_2=Limits_VDCreg(2), Kp_Ireg=Kp_Ireg, Ki_Ireg=Ki_Ireg, Limits_Ireg=Limits_Ireg, Rff=Rff, Lff=Lff, Kp_CCSC=Kp_CCSC, Ki_CCSC=Ki_CCSC}
      mask prompts: Ts "Sample time:"; Fnom "Fundamental frequency (Hz):"; Fn_filter "Natural frequency fn (Hz):"; Zeta_filter "Damping ratio Zeta"; Kp_Preg "Proportional (P):"; Ki_Preg "Integral (I):"; Limits_Preg_1 "Upper limit:"; Limits_Preg_2 "Lower limit:"; Kp_Qreg "Proportional (P):"; Ki_Qreg "Integral (I):"; Limits_Qreg_1 "Upper limit:"; Limits_Qreg_2 "Lower limit:"; Kp_VDCreg "Proportional (P):"; Ki_VDCreg "Integral (I):"; Limits_VDCreg_1 "Upper limit:"; Limits_VDCreg_2 "Lower limit:"; Kp_Ireg "Proportional (P):"; Ki_Ireg "Integral (I):"; Limits_Ireg "Output limits:"; Kp_CCSC "Proportional (P):"; Ki_CCSC "Integral (I):"
      mask DialogControl Container6 Prompt: General
      mask DialogControl Container14 Prompt: Filter
      mask DialogControl Container14_copy Prompt: Active power regulator
      mask DialogControl Container14_copy_copy Prompt: Reactive power regulator
      mask DialogControl Container14_copy_copy_copy Prompt: DC voltage regulator
      mask DialogControl Container14_copy_copy_copy_copy Prompt: Current regulator
      mask DialogControl Container14_copy_copy_copy_copy_copy Prompt: CCSC
  V->pu2 : Gain  Gain=1/Vb_ac  SaturateOnIntegerOverflow=on  OutDataTypeStr=Inherit: Same as input  ParamDataTypeStr=Inherit: Same as input
  abc to dq0 : spsabctodq0Lib/abc to dq0  Alignment=90 degrees behind phase A axis
  abc to dq1 : spsabctodq0Lib/abc to dq0  Alignment=90 degrees behind phase A axis
  "{m_dq1}" : Outport  VectorParamsAs1DForOutWhenUnconnected=off
  "{m_dq2}" : Outport  Port=2  VectorParamsAs1DForOutWhenUnconnected=off
  wires:
  Subsystem1/1(m_dq1) -> "{m_dq1}"/1
  Vsec/1 -> V->pu2/1
  abc to dq1/1 -> Selector5/1
  Vdc/1 -> I->pu9/1
  Iconv/1 -> I->pu2/1
  I->pu2/1 -> abc to dq1/1
  Park Transform4/1 -> Selector2/1
  I->pu9/1 -> Subsystem1/1(Vdc)
  Gain9/1 -> Park Transform4/2
  wt/1 -> abc to dq0/2, Gain9/1, abc to dq1/2
  Subsystem1/2(m_dq2) -> "{m_dq2}"/1
  abc to dq0/1 -> Selector4/1
  Selector5/1 -> Subsystem1/3(Iconv_dq1)
  Selector4/1 -> Subsystem1/2(Vs_dq1)
  V->pu2/1 -> abc to dq0/1
  Idiff/1 -> I->pu4/1
  Selector2/1 -> Subsystem1/4(Id_dq2)
  I->pu4/1 -> Park Transform4/1
  [PQreg_On] -> Subsystem1/5(PQreg_On)
  [VDCreg_On] -> Subsystem1/6(VDCreg_On)
  [Vdc_ref] -> Subsystem1/7(Vdc_ref)
  [PSCC_On] -> Subsystem1/8(PQreg_On1)

== system HVDC_MMC1_EMT/Voltage source ==
  In1 : Inport
  Controlled Voltage Source : spsControlledVoltageSourceLib/Controlled Voltage Source  Initialize=on  Source_Type=AC  Amplitude=0  Phase=0  Frequency=0  Measurements=None
  Controlled Voltage Source6 : spsControlledVoltageSourceLib/Controlled Voltage Source  Initialize=on  Source_Type=AC  Amplitude=0  Phase=0  Frequency=0  Measurements=None
  Controlled Voltage Source7 : spsControlledVoltageSourceLib/Controlled Voltage Source  Initialize=on  Source_Type=AC  Amplitude=0  Phase=0  Frequency=0  Measurements=None
  Demux9 : Demux  Outputs=3
  Ground : spsGroundLib/Ground  LConnTagsString=a
  a : PMIOPort  Side=Right
  b : PMIOPort  Port=2  Side=Right
  c : PMIOPort  Port=3  Side=Right
  wires:
  In1/1 -> Demux9/1
  Demux9/1 -> Controlled Voltage Source/1
  Demux9/2 -> Controlled Voltage Source6/1
  Demux9/3 -> Controlled Voltage Source7/1
  connections:
  Ground/LConn1 -- Controlled Voltage Source6/LConn1 -- Controlled Voltage Source/LConn1 -- Controlled Voltage Source7/LConn1
  Controlled Voltage Source7/RConn1 -- c/RConn1
  Controlled Voltage Source6/RConn1 -- b/RConn1
  Controlled Voltage Source/RConn1 -- a/RConn1

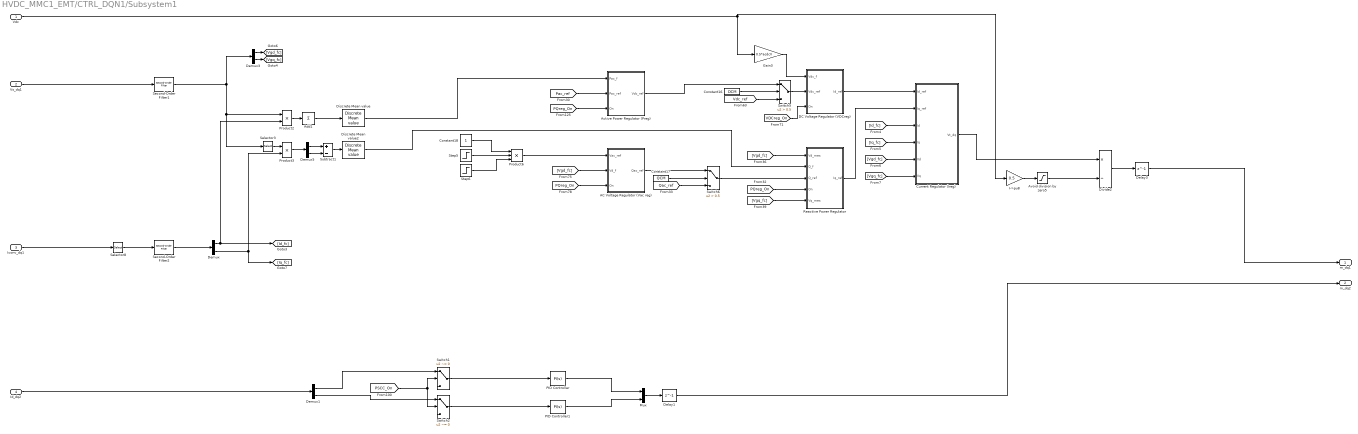
== system HVDC_MMC1_EMT/CTRL_DQN1/Subsystem1 ==
  Vdc : Inport
  Vs_dq1 : Inport  Port=2
  Iconv_dq1 : Inport  Port=3
  Id_dq2 : Inport  Port=4
  AC Voltage Regulator (Vac reg) : Subsystem
  Active Power Regulator (Preg) : Subsystem
  Add1 : Sum  Inputs=1
  Avoid division by zero5 : Saturate  UpperLimit=10*acdcV  LowerLimit=0.5/acdcV  ZeroCross=off
  Constant16 : Constant  Value=DCM
  Constant17 : Constant  Value=QCM
  Constant18 : Constant
  Current Regulator (Ireg) : Subsystem
  DC Voltage Regulator (VDCreg) : Subsystem
  Delay1 : Delay  DelayLength=1
  Delay3 : Delay  DelayLength=1
  Demux{,1,3,5} (4 alike) : Demux  Outputs=2
  Discrete Mean value : powerlib_extras/Discrete Measurements/Discrete  Mean value  Freq=Fnom  Vinit=0  Ts=Ts
  Discrete Mean value2 : powerlib_extras/Discrete Measurements/Discrete  Mean value  Freq=Fnom  Vinit=0  Ts=Ts
  Divide2 : Product  Inputs=*/
  Gain3 : Gain  Gain=0.5*acdcV
  I->pu8 : Gain  Gain=0.5  SaturateOnIntegerOverflow=on  OutDataTypeStr=Inherit: Same as input  ParamDataTypeStr=Inherit: Same as input
  Mux : Mux  Inputs=2
  PID Controller : slpidlib/PID Controller  Controller=PI  Form=Parallel  TimeDomain=Continuous-time  UseExternalTs=off  SampleTime=-1  IntegratorMethod=Forward Euler  FilterMethod=Forward Euler  ControllerParametersSource=internal  P=Kp_CCSC  I=Ki_CCSC  UseKiTs=off  D=0  N=100  UseFilter=on  TunerSelectOption=Transfer Function Based (PID Tuner App)  InitialConditionSource=internal  InitialConditionForIntegrator=0  InitialConditionForFilter=0  DifferentiatorICPrevScaledInput=0  ExternalReset=none  TrackingMode=off  Kt=1  LimitOutput=off  SatLimitsSource=internal  UpperSaturationLimit=inf  LowerSaturationLimit=-inf  LinearizeAsGain=on  AntiWindupMode=none  Kb=1  LimitIntegrator=off  UpperIntegratorSaturationLimit=inf  LowerIntegratorSaturationLimit=-inf  POutMin=[]  POutMax=[]  IOutMin=[]  IOutMax=[]  DOutMin=[]  DOutMax=[]  NOutMin=[]  NOutMax=[]  SumOutMin=[]  SumOutMax=[]  SaturationOutMin=[]  SaturationOutMax=[]  PParamMin=[]  PParamMax=[]  IParamMin=[]  IParamMax=[]  DParamMin=[]  DParamMax=[]  NParamMin=[]  NParamMax=[]  KbParamMin=[]  KbParamMax=[]  KtParamMin=[]  KtParamMax=[]  KbOutMin=[]  KbOutMax=[]  KtOutMin=[]  KtOutMax=[]  IntegratorOutMin=[]  IntegratorOutMax=[]  FilterOutMin=[]  FilterOutMax=[]  SumI1OutMin=[]  SumI1OutMax=[]  SumI2OutMin=[]  SumI2OutMax=[]  SumI3OutMin=[]  SumI3OutMax=[]  SumI4OutMin=[]  SumI4OutMax=[]  SumDOutMin=[]  SumDOutMax=[]  DifferentiatorOutMin=[]  DifferentiatorOutMax=[]  FilterDiffOutCoefMin=[]  FilterDiffOutCoefMax=[]  ReciprocalOutMin=[]  ReciprocalOutMax=[]  SumDenOutMin=[]  SumDenOutMax=[]  SumNumOutMin=[]  SumNumOutMax=[]  DivideOutMin=[]  DivideOutMax=[]  UdiffTsProdOutMin=[]  UdiffTsProdOutMax=[]  NTsProdOutMin=[]  NTsProdOutMax=[]  UintegralTsProdOutMin=[]  UintegralTsProdOutMax=[]  UngainTsProdOutMin=[]  UngainTsProdOutMax=[]  ClampingZeroOutDataTypeStr=Inherit: Inherit via back propagation  ClampingZeroOutMin=[]  ClampingZeroOutMax=[]  FilterDenConstantOutDataTypeStr=Inherit: Inherit via back propagation  FilterDenConstantOutMin=[]  FilterDenConstantOutMax=[]  PCopyOutDataTypeStr=Inherit: Inherit via back propagation  PCopyOutMin=[]  PCopyOutMax=[]  NCopyOutDataTypeStr=Inherit: Inherit via back propagation  NCopyOutMin=[]  NCopyOutMax=[]  IntegratorContinuousStateAttributes=''  IntegratorStateMustResolveToSignalObject=off  IntegratorRTWStateStorageClass=Auto  FilterContinuousStateAttributes=''  FilterStateMustResolveToSignalObject=off  FilterRTWStateStorageClass=Auto  ParallelPVariant=InternalParameters  IdealPVariant=Disabled  IVariant=InternalParameters  DVariant=Disabled  IntegratorVariant=Continuous  SatVariant=Disabled  AWVariant=Passthrough  PCopyVariant=Disabled  TRVariant=Disabled  FdbkBlocksVariant=Forward  IdealPFdbkVariant=Disabled  SatFdbkVariant=Disabled  DerivativeFilterVariant=Disabled  NVariant=Disabled  NCopyVariant=Disabled_SignalSpec  FilterICVariant=Disabled  IntegratorICVariant=InternalICs  ExternalResetVariant=Disabled  TRSumVariant=Passthrough  SumFdbkVariant=Disabled  SumVariant=Sum_PI  TsampFilterVariant=InternalTs  TsampNgainVariant=Passthrough  TsampIntegralVariant=Disabled_SignalSpec  ExternalSaturationOutDataTypeStr=Inherit: Same as second input
  PID Controller1 : slpidlib/PID Controller  Controller=PI  Form=Parallel  TimeDomain=Continuous-time  UseExternalTs=off  SampleTime=-1  IntegratorMethod=Forward Euler  FilterMethod=Forward Euler  ControllerParametersSource=internal  P=Kp_CCSC  I=Ki_CCSC  UseKiTs=off  D=0  N=100  UseFilter=on  TunerSelectOption=Transfer Function Based (PID Tuner App)  InitialConditionSource=internal  InitialConditionForIntegrator=0  InitialConditionForFilter=0  DifferentiatorICPrevScaledInput=0  ExternalReset=none  TrackingMode=off  Kt=1  LimitOutput=off  SatLimitsSource=internal  UpperSaturationLimit=inf  LowerSaturationLimit=-inf  LinearizeAsGain=on  AntiWindupMode=none  Kb=1  LimitIntegrator=off  UpperIntegratorSaturationLimit=inf  LowerIntegratorSaturationLimit=-inf  POutMin=[]  POutMax=[]  IOutMin=[]  IOutMax=[]  DOutMin=[]  DOutMax=[]  NOutMin=[]  NOutMax=[]  SumOutMin=[]  SumOutMax=[]  SaturationOutMin=[]  SaturationOutMax=[]  PParamMin=[]  PParamMax=[]  IParamMin=[]  IParamMax=[]  DParamMin=[]  DParamMax=[]  NParamMin=[]  NParamMax=[]  KbParamMin=[]  KbParamMax=[]  KtParamMin=[]  KtParamMax=[]  KbOutMin=[]  KbOutMax=[]  KtOutMin=[]  KtOutMax=[]  IntegratorOutMin=[]  IntegratorOutMax=[]  FilterOutMin=[]  FilterOutMax=[]  SumI1OutMin=[]  SumI1OutMax=[]  SumI2OutMin=[]  SumI2OutMax=[]  SumI3OutMin=[]  SumI3OutMax=[]  SumI4OutMin=[]  SumI4OutMax=[]  SumDOutMin=[]  SumDOutMax=[]  DifferentiatorOutMin=[]  DifferentiatorOutMax=[]  FilterDiffOutCoefMin=[]  FilterDiffOutCoefMax=[]  ReciprocalOutMin=[]  ReciprocalOutMax=[]  SumDenOutMin=[]  SumDenOutMax=[]  SumNumOutMin=[]  SumNumOutMax=[]  DivideOutMin=[]  DivideOutMax=[]  UdiffTsProdOutMin=[]  UdiffTsProdOutMax=[]  NTsProdOutMin=[]  NTsProdOutMax=[]  UintegralTsProdOutMin=[]  UintegralTsProdOutMax=[]  UngainTsProdOutMin=[]  UngainTsProdOutMax=[]  ClampingZeroOutDataTypeStr=Inherit: Inherit via back propagation  ClampingZeroOutMin=[]  ClampingZeroOutMax=[]  FilterDenConstantOutDataTypeStr=Inherit: Inherit via back propagation  FilterDenConstantOutMin=[]  FilterDenConstantOutMax=[]  PCopyOutDataTypeStr=Inherit: Inherit via back propagation  PCopyOutMin=[]  PCopyOutMax=[]  NCopyOutDataTypeStr=Inherit: Inherit via back propagation  NCopyOutMin=[]  NCopyOutMax=[]  IntegratorContinuousStateAttributes=''  IntegratorStateMustResolveToSignalObject=off  IntegratorRTWStateStorageClass=Auto  FilterContinuousStateAttributes=''  FilterStateMustResolveToSignalObject=off  FilterRTWStateStorageClass=Auto  ParallelPVariant=InternalParameters  IdealPVariant=Disabled  IVariant=InternalParameters  DVariant=Disabled  IntegratorVariant=Continuous  SatVariant=Disabled  AWVariant=Passthrough  PCopyVariant=Disabled  TRVariant=Disabled  FdbkBlocksVariant=Forward  IdealPFdbkVariant=Disabled  SatFdbkVariant=Disabled  DerivativeFilterVariant=Disabled  NVariant=Disabled  NCopyVariant=Disabled_SignalSpec  FilterICVariant=Disabled  IntegratorICVariant=InternalICs  ExternalResetVariant=Disabled  TRSumVariant=Passthrough  SumFdbkVariant=Disabled  SumVariant=Sum_PI  TsampFilterVariant=InternalTs  TsampNgainVariant=Passthrough  TsampIntegralVariant=Disabled_SignalSpec  ExternalSaturationOutDataTypeStr=Inherit: Same as second input
  Product2 : Product  RndMeth=Zero
  Product3 : Product  RndMeth=Zero
  Product6 : Product  Inputs=3
  Reactive Power Regulator : Subsystem
  Second-Order Filter1 : spsSecondOrderFilterLib/Second-Order Filter  FilterType=Lowpass  Fo=Fn_filter  Zeta=Zeta_filter  Ts=Ts  Initialize=off  Vac_Init="[0,  0,  60]"  Vdc_Init=0  PlotResponse=off  FreqRange=[0, 500, 1]
  Second-Order Filter2 : spsSecondOrderFilterLib/Second-Order Filter  FilterType=Lowpass  Fo=Fn_filter  Zeta=Zeta_filter  Ts=Ts  Initialize=off  Vac_Init="[0,  0,  60]"  Vdc_Init=0  PlotResponse=off  FreqRange=[0, 500, 1]
  Selector3 : Selector  InputPortWidth=2  IndexOptions=Index vector (dialog)  Indices=[2 1]  OutputSizes=1
  Selector8 : Selector  InputPortWidth=2  IndexOptions=Index vector (dialog)  Indices=[1 2]  OutputSizes=1
  Step5 : Step  Time=7  Before=1  After=0.99  SampleTime=0
  Step6 : Step  Time=9  Before=1  After=1.01/0.99  SampleTime=0
  Subtract1 : Sum  Inputs=+-
  Switch1 : Switch  Criteria=u2 ~= 0  Threshold=0.5  OutDataTypeStr=double  SaturateOnIntegerOverflow=off  InputSameDT=off
  Switch2 : Switch  Criteria=u2 ~= 0  Threshold=0.5  OutDataTypeStr=double  SaturateOnIntegerOverflow=off  InputSameDT=off
  Switch5 : Switch  Criteria=u2 > Threshold  Threshold=0.5  OutDataTypeStr=double  SaturateOnIntegerOverflow=off  InputSameDT=off
  Switch6 : Switch  Criteria=u2 > Threshold  Threshold=0.5  OutDataTypeStr=double  SaturateOnIntegerOverflow=off  InputSameDT=off
  m_dq1 : Outport
  m_dq2 : Outport  Port=2
  wires:
  DC Voltage Regulator (VDCreg)/1(Id_ref) -> Current Regulator (Ireg)/1(Id_ref)
  Second-Order Filter2/1 -> Demux/1
  Demux/2 -> Product3/2, [Iq_fc]
  Active Power Regulator (Preg)/1(Vdc_ref) -> Switch5/1
  [PQreg_On] -> AC Voltage Regulator (Vac reg)/3(On)
  Vdc/1 -> I->pu8/1, Gain3/1
  PID Controller1/1 -> Mux/2
  Mux/1 -> Delay1/1
  Demux3/1 -> [Vgd_fc]
  [Vgq_fc] -> Reactive Power Regulator/5(Vq_mes)
  [Vgq_fc] -> Current Regulator (Ireg)/6(Vq)
  Add1/1 -> Discrete Mean value/1
  Switch6/1 -> Reactive Power Regulator/3(Q_ref)
  Product6/1 -> AC Voltage Regulator (Vac reg)/1(Vac_ref)
  Product2/1 -> Add1/1
  Discrete Mean value/1 -> Active Power Regulator (Preg)/1(Pac_f)
  Current Regulator (Ireg)/1(Vt_dq) -> Divide2/1
  Demux5/1 -> Subtract1/1
  [Iq_fc] -> Current Regulator (Ireg)/4(Iq)
  Divide2/1 -> Delay3/1
  I->pu8/1 -> Avoid division by zero5/1
  Constant18/1 -> Product6/1
  [Qac_ref] -> Switch6/3
  Selector3/1 -> Product3/1
  [PQreg_On] -> Reactive Power Regulator/4(On)
  Gain3/1 -> DC Voltage Regulator (VDCreg)/1(Vdc_f)
  Constant17/1 -> Switch6/2
  [Vgd_fc] -> AC Voltage Regulator (Vac reg)/2(Vd_f)
  Demux3/2 -> [Vgq_fc]
  Constant16/1 -> Switch5/2
  Reactive Power Regulator/1(Iq_ref) -> Current Regulator (Ireg)/2(Iq_ref)
  [VDCreg_On] -> DC Voltage Regulator (VDCreg)/3(On)
  Switch5/1 -> DC Voltage Regulator (VDCreg)/2(Vdc_ref)
  [Vgd_fc] -> Reactive Power Regulator/1(Vd_mes)
  [PSCC_On] -> Switch1/2, Switch2/2
  Subtract1/1 -> Discrete Mean value2/1
  Product3/1 -> Demux5/1
  Avoid division by zero5/1 -> Divide2/2
  Step6/1 -> Product6/3
  Demux5/2 -> Subtract1/2
  AC Voltage Regulator (Vac reg)/1(Qac_ref) -> Switch6/1
  Step5/1 -> Product6/2
  Demux/1 -> [Id_fc], Product2/2
  [Pac_ref] -> Active Power Regulator (Preg)/2(Pac_ref)
  [Id_fc] -> Current Regulator (Ireg)/3(Id)
  Second-Order Filter1/1 -> Selector3/1, Product2/1, Demux3/1
  PID Controller/1 -> Mux/1
  Selector8/1 -> Second-Order Filter2/1
  [PQreg_On] -> Active Power Regulator (Preg)/3(On)
  [Vgd_fc] -> Current Regulator (Ireg)/5(Vd)
  Discrete Mean value2/1 -> Reactive Power Regulator/2(Q_f)
  [Vdc_ref] -> Switch5/3
  Delay3/1 -> m_dq1/1
  Vs_dq1/1 -> Second-Order Filter1/1
  Iconv_dq1/1 -> Selector8/1
  Demux1/1 -> Switch1/1
  Demux1/2 -> Switch2/1
  Id_dq2/1 -> Demux1/1
  Switch1/1 -> PID Controller/1
  Switch2/1 -> PID Controller1/1
  Delay1/1 -> m_dq2/1
